simulink model "chap11_2sim"  (R2015a)
settings: Solver=ode45  StartTime=0.0  StopTime=10  RelTol=1e-3
settings Model: Creator=zhr  LastModifiedBy=IT

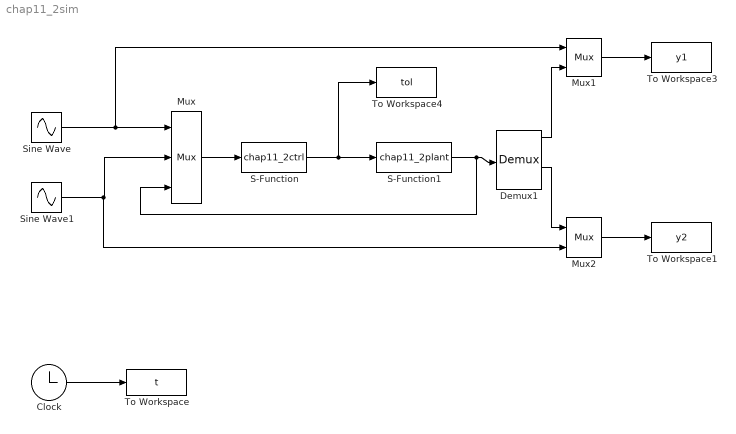
== system chap11_2sim ==
  Clock : Clock
  Demux1 : Demux
  Mux : Mux  Inputs=3
  Mux1 : Mux  Inputs=2
  Mux2 : Mux  Inputs=2
  S-Function : S-Function  FunctionName=chap11_2ctrl
  S-Function1 : S-Function  FunctionName=chap11_2plant
  Sine Wave : Sin  Bias=0.5  SampleTime=0
  Sine Wave1 : Sin  SampleTime=0
  To Workspace : ToWorkspace  VariableName=t  SampleTime=-1
  To Workspace1 : ToWorkspace  VariableName=y2  SampleTime=-1
  To Workspace3 : ToWorkspace  VariableName=y1  SampleTime=-1
  To Workspace4 : ToWorkspace  VariableName=tol  SampleTime=-1
  wires:
  Clock/1 -> To Workspace/1
  Mux/1 -> S-Function/1
  S-Function/1 -> To Workspace4/1, S-Function1/1
  S-Function1/1 -> Mux/3, Demux1/1
  Sine Wave/1 -> Mux1/1, Mux/1
  Demux1/3 -> Mux2/1
  Demux1/1 -> Mux1/2
  Sine Wave1/1 -> Mux2/2, Mux/2
  Mux2/1 -> To Workspace1/1
  Mux1/1 -> To Workspace3/1
